simulink model "mealy_moore"  (R2016a)
settings: Solver=FixedStepDiscrete  SolverMode=SingleTasking  StartTime=0.0  StopTime=10  RelTol=1e-3
libraries: hdlsllib x2
settings Model: DataTypeOverride=Off  Creator=sande  LastModifiedBy=sande
settings SolverCC: AutoInsertRateTranBlk=on
settings DataIOCC: LimitDataPoints=on  SaveFormat=Array  SaveOutput=off  SaveTime=off
settings OptimizationCC: BlockReduction=off  ConditionallyExecuteInputs=off  DefaultParameterBehavior=Inlined  UseDivisionForNetSlopeComputation=UseDivisionForReciprocalsOfIntegersOnly  UseFloatMulNetSlope=on  InlineInvariantSignals=on  EnhancedBackFolding=on  EfficientFloat2IntCast=on  OptimizeModelRefInitCode=on  LifeSpan=1
settings DebuggingCC: AlgebraicLoopMsg=error  SolverPrmCheckMsg=warning  InheritedTsInSrcMsg=none  SingleTaskRateTransMsg=error  AllowSymbolicDim=off  StrictBusMsg=ErrorOnBusTreatedAsVector  NonBusSignalsTreatedAsBus=error
settings HardwareCC: ProdBitPerPointer=32  ProdLargestAtomicFloat=None  ProdIntDivRoundTo=Undefined  ProdEndianess=Unspecified  ProdWordSize=32  ProdHWDeviceType=ASIC/FPGA->ASIC/FPGA  TargetBitPerPointer=64  TargetLongLongMode=on  TargetIntDivRoundTo=Zero  TargetEndianess=LittleEndian  TargetWordSize=64  TargetHWDeviceType=MATLAB Host  ProdEqTarget=off
settings ModelReferenceCC: PropagateSignalLabelsOutOfModel=off
settings RTWCC: SystemTargetFile=ert.tlc  GenCodeOnly=on  PackageGeneratedCodeAndArtifacts=on  TemplateMakefile=ert_default_tmf  GenerateReport=on  BuildConfiguration=Faster Runs  IncludeHyperlinkInReport=on  LaunchReport=on  TargetLang=C++  GenerateTraceInfo=on  GenerateTraceReport=on  GenerateTraceReportSl=on  GenerateTraceReportSf=on  GenerateTraceReportEml=on  GenerateCodeMetricsReport=on
settings ERTTargetCC: GenerateSampleERTMain=on  CombineSignalStateStructs=on  SuppressErrorStatus=on  MultiInstanceERTCode=on  CodeInterfacePackaging=C++ class  InlinedParameterPlacement=NonHierarchical  RootIOFormat=Structure reference  ERTCustomFileTemplate=example_file_process.tlc  ConvertIfToSwitch=off  SuppressUnreachableDefaultCases=off
settings ConfigComp: CovModelRefEnable=Off  CovSFcnEnable=off

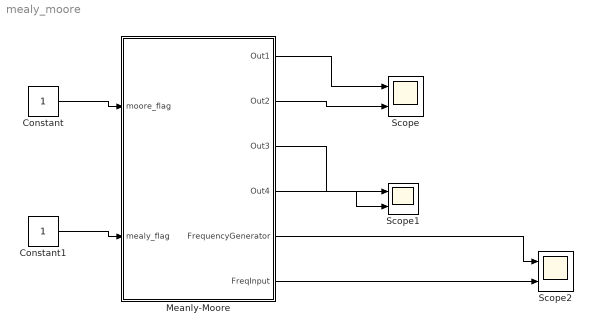
== system mealy_moore ==
  Constant : Constant  OutDataTypeStr=boolean  SampleTime=1
  Constant1 : Constant  OutDataTypeStr=boolean  SampleTime=1
  Meanly-Moore : Subsystem
  Scope : Scope  NumInputPorts=2
  Scope1 : Scope  NumInputPorts=2
  Scope2 : Scope  NumInputPorts=2
  wires:
  Constant/1 -> Meanly-Moore/1(moore_flag)
  Constant1/1 -> Meanly-Moore/2(mealy_flag)
  Meanly-Moore/1(Out1) -> Scope/1
  Meanly-Moore/2(Out2) -> Scope/2
  Meanly-Moore/3(Out3) -> Scope1/1
  Meanly-Moore/4(Out4) -> Scope1/2
  Meanly-Moore/5(FrequencyGenerator) -> Scope2/1
  Meanly-Moore/6(FreqInput) -> Scope2/2

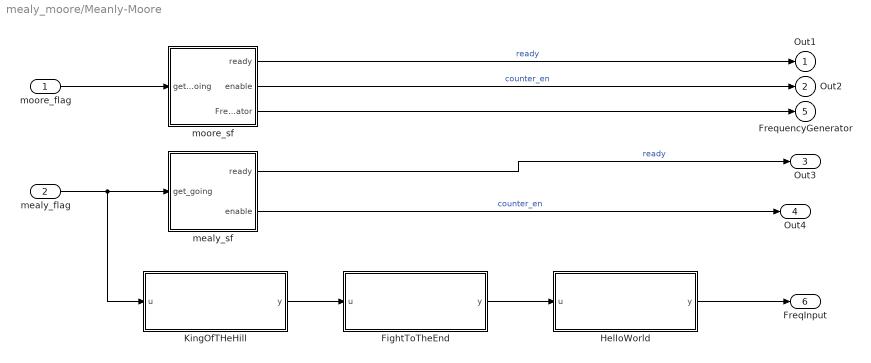
== system mealy_moore/Meanly-Moore ==
  moore_flag : Inport
  mealy_flag : Inport  Port=2
  FightToTheEnd : MATLAB Function  TreatAsAtomicUnit=on
  HelloWorld : MATLAB Function  TreatAsAtomicUnit=on
  KingOfTHeHill : MATLAB Function  TreatAsAtomicUnit=on
  mealy_sf : Subsystem
  moore_sf : Subsystem
  Out1 : Outport
  Out2 : Outport  Port=2
  Out3 : Outport  Port=3
  Out4 : Outport  Port=4
  FrequencyGenerator : Outport  Port=5
  FreqInput : Outport  Port=6
  wires:
  mealy_flag/1 -> mealy_sf/1(get_going), KingOfTHeHill/1(u)
  mealy_sf/2(enable) -> Out4/1  "counter_en"
  moore_sf/1(ready) -> Out1/1  "ready"
  moore_flag/1 -> moore_sf/1(get_going)
  moore_sf/2(enable) -> Out2/1  "counter_en"
  mealy_sf/1(ready) -> Out3/1  "ready"
  moore_sf/3(FrequencyGenerator) -> FrequencyGenerator/1
  FightToTheEnd/1(y) -> HelloWorld/1(u)
  HelloWorld/1(y) -> FreqInput/1
  KingOfTHeHill/1(y) -> FightToTheEnd/1(u)

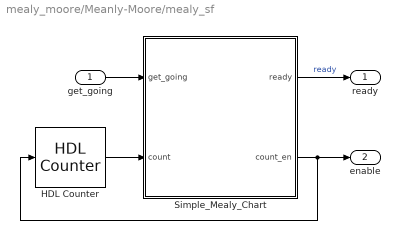
== system mealy_moore/Meanly-Moore/mealy_sf ==
  get_going : Inport
  HDL Counter : hdlsllib/HDL Operations/HDL Counter  CountType=Count limited  CountInit=0  CountStep=1  CountMax=25  CountFromType=Initial value  CountFrom=0  CountResetPort=off  CountLoadPort=off  CountEnbPort=on  CountDirPort=off  CountDataType=Unsigned  CountWordLen=8  CountFracLen=0  CountSampTime=1
  Simple_Mealy_Chart : Stateflow chart  TreatAsAtomicUnit=on
  ready : Outport
  enable : Outport  Port=2
  wires:
  get_going/1 -> Simple_Mealy_Chart/1(get_going)
  Simple_Mealy_Chart/1(ready) -> ready/1  "ready"
  Simple_Mealy_Chart/2(count_en) -> HDL Counter/1, enable/1
  HDL Counter/1 -> Simple_Mealy_Chart/2(count)

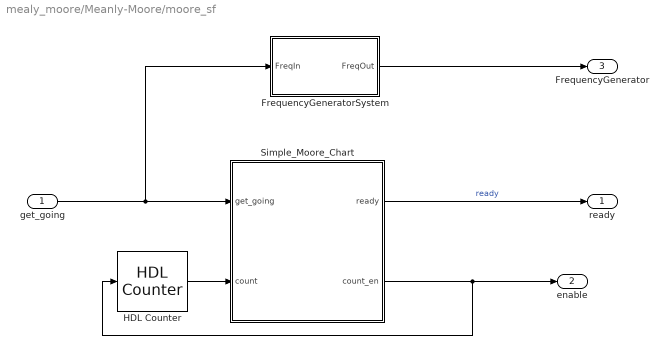
== system mealy_moore/Meanly-Moore/moore_sf ==
  get_going : Inport
  FrequencyGeneratorSystem : Subsystem
  HDL Counter : hdlsllib/HDL Operations/HDL Counter  CountType=Count limited  CountInit=0  CountStep=1  CountMax=25  CountFromType=Initial value  CountFrom=0  CountResetPort=off  CountLoadPort=off  CountEnbPort=on  CountDirPort=off  CountDataType=Unsigned  CountWordLen=8  CountFracLen=0  CountSampTime=1
  Simple_Moore_Chart : Stateflow chart  TreatAsAtomicUnit=on
  ready : Outport
  enable : Outport  Port=2
  FrequencyGenerator : Outport  Port=3
  wires:
  Simple_Moore_Chart/2(count_en) -> HDL Counter/1, enable/1
  HDL Counter/1 -> Simple_Moore_Chart/2(count)
  Simple_Moore_Chart/1(ready) -> ready/1  "ready"
  get_going/1 -> FrequencyGeneratorSystem/1(FreqIn), Simple_Moore_Chart/1(get_going)
  FrequencyGeneratorSystem/1(FreqOut) -> FrequencyGenerator/1

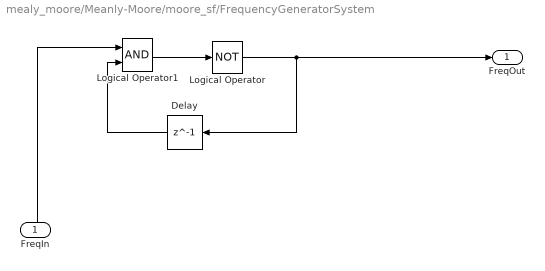
== system mealy_moore/Meanly-Moore/moore_sf/FrequencyGeneratorSystem ==
  FreqIn : Inport
  Delay : Delay  DelayLength=1  InitialCondition=1
  Logical Operator : Logic  Operator=NOT  AllPortsSameDT=off  OutDataTypeStr=boolean
  Logical Operator1 : Logic  AllPortsSameDT=off  OutDataTypeStr=boolean
  FreqOut : Outport
  wires:
  Logical Operator1/1 -> Logical Operator/1
  Logical Operator/1 -> FreqOut/1, Delay/1
  Delay/1 -> Logical Operator1/2
  FreqIn/1 -> Logical Operator1/1

== stateflow chart mealy_moore/Meanly-Moore/moore_sf/Simple_Moore_Chart ==
  settings: stateMachineType=MOORE_MACHINE  initializeOutput=1
  state IDLE
    ready = true;
    count_en = false;
  state COUNTING
    ready = false;
    count_en = true;
  (default) -> IDLE
  COUNTING -> IDLE : [(count) == max_count]
  IDLE -> COUNTING : [get_going == true]
  data: get_going input boolean; count input =0; ready output boolean =true; count_en output boolean; max_count constant fixdt(0,5,0) =25

== stateflow chart mealy_moore/Meanly-Moore/mealy_sf/Simple_Mealy_Chart ==
  settings: stateMachineType=MEALY_MACHINE  executeAtInitialization=1
  state IDLE
  state COUNTING
  (default) -> IDLE
  COUNTING -> IDLE : [count == max_count]...
      | {ready = true;...
      | count_en = false;}
  IDLE -> COUNTING : [get_going == true]...
      | {ready = false;...
      |  count_en = true;}
  data: get_going input boolean; count input uint8 =0; ready output boolean =true; count_en output boolean; max_count constant uint8 =25

== matlab function mealy_moore/Meanly-Moore/KingOfTHeHill ==
  data: u input; y output
function y = fcn(u)
%#codegen

y = u;

== matlab function mealy_moore/Meanly-Moore/FightToTheEnd ==
  data: u input; y output
function y = fcn(u)
%#codegen

y = u;

== matlab function mealy_moore/Meanly-Moore/HelloWorld ==
  data: u input; y output
function y = fcn(u)
%#codegen

y = u;
